simulink model "Controller_Exp"  (R2016a)
settings: Solver=ode4  StartTime=0.0  StopTime=Inf  FixedStep=Ts  RelTol=1e-3
undefined symbols (not defined in the file or in its folder): A_lpf_velocity, B1_lpf_velocity, B2_lpf_velocity, Calibration, commanded_u, GearOffsets, IMUTorsoOffsets, MedullaCommand, ResetDAQ, sample_time, TorsoCOMOffsets, Ts
libraries: xpcethercatlib x188, simulink x37, slrtlib x11, ControllerLibrary x2, dspswit3 x1
(part 4 of 4)

== system Controller_Exp/DAQ/DAQ_sub/Subsystem/EtherCATRobotMicrostrain/LegElmo_2R/Subsystem1/EnableControlWord ==
  Action Port : ActionPort  ActionType=case
  Constant : Constant  Value=15  OutDataTypeStr=uint16
  ControlWord : Outport
  wires:
  Constant/1 -> ControlWord/1

== system Controller_Exp/DAQ/DAQ_sub/Subsystem/EtherCATRobotMicrostrain/LegElmo_2R/Subsystem1/FaultReset ==
  Action Port : ActionPort  ActionType=case
  Constant : Constant  Value=128  OutDataTypeStr=uint16
  ControlWord : Outport
  wires:
  Constant/1 -> ControlWord/1

== system Controller_Exp/DAQ/DAQ_sub/Subsystem/EtherCATRobotMicrostrain/LegElmo_2R/Subsystem1/NothingControlWord ==
  Action Port : ActionPort  ActionType=default
  Constant : Constant  Value=0  OutDataTypeStr=uint16
  ControlWord : Outport
  wires:
  Constant/1 -> ControlWord/1

== system Controller_Exp/DAQ/DAQ_sub/Subsystem/EtherCATRobotMicrostrain/LegElmo_2R/Subsystem1/ShutdownControlWord ==
  Action Port : ActionPort  ActionType=case
  Constant : Constant  Value=6  OutDataTypeStr=uint16
  ControlWord : Outport
  wires:
  Constant/1 -> ControlWord/1

== matlab function Controller_Exp/DAQ/DAQ_sub/Subsystem/EstimateOrientation ==
  data: DeltaAngle input; Acceleration input; Status input; Sequence input; Reset input; Rk output; wk output; Rkm1 input; wkm1 input; Akm1 input; Ak output; Seqkm1 input; Seqk output; ValidStates output
function [Rk, wk, Ak, Seqk, ValidStates] = fcn(DeltaAngle,Acceleration,Status,Sequence,Reset,Rkm1,wkm1,Akm1,Seqkm1) %#codegen
    [Rk, wk, Ak, Seqk, ValidStates] = estimateOrientation(DeltaAngle,Acceleration,Rkm1,wkm1,Akm1,Status,Sequence,Seqkm1,Reset);
end

== matlab function Controller_Exp/DAQ/DAQ_sub/Subsystem/ComputeEulerAngles ==
  data: RkIn input; wk input; RCal input; Reset input; R0In input; ZYX output size=3; dZYX output size=3; Rk output; R0 output; YawRolloverIn input; YawRollover output
function [ZYX, dZYX, Rk, R0, YawRollover] = fcn(RkIn, wk, RCal, Reset, R0In, YawRolloverIn) %#codegen
    % Convert from IMU frame to robot frame and compute Euler angles. The
    % yaw angle is zeroed whenever (Reset) is true.
        
    if (Reset)
        % Compute the rotation matrix which zeroes the initial yaw
        qT0 = M_to_ZYX(RkIn*RCal);
        R0  = Rz(-qT0(1));
    else
        R0 = R0In;
    end
    
    % Transform from IMU to robot frame and zero initial yaw
    Rk = R0*RkIn*RCal;
    
    % Convert Rk to ZYX Euler angles
    ZYX = M_to_ZYX(Rk);
    
    % Unroll yaw
    YawRolloverCount = YawRolloverIn(1);
    PreviousYaw      = YawRolloverIn(2);
    CurrentYaw       = ZYX(1);
    YawRolloverCount = YawRolloverCount + getYawRollover(CurrentYaw, PreviousYaw);
    YawRollover      = [YawRolloverCount; CurrentYaw];
    ZYX(1)           = ZYX(1) + 2*pi*YawRolloverCount;
    
    % Compute Euler angle derivatives
    qzT = ZYX(1);
    qyT = ZYX(2);
    
    if cos(qyT)>1e-3
        dZYX = [0 -sin(qzT) cos(qzT)*cos(qyT); 0 cos(qzT) sin(qzT)*cos(qyT); 1 0 -sin(qyT)]\(R0*RkIn*wk);
    else
        dZYX = [0; 0; 0];
    end
end

function R = Rz(t)
    R = [cos(t) -sin(t) 0; sin(t) cos(t) 0; 0 0 1];
end

function Rollover = getYawRollover(CurrentYaw, PreviousYaw)
    % Determine if a rollover has occurred on yaw angle If a rollover is
    % detected, the output Rollover is either +1 or -1, depending on the
    % direction of the rollover.
  
    if (PreviousYaw>0 && CurrentYaw < (PreviousYaw-pi))
        Rollover = 1;
    elseif (PreviousYaw<0 && CurrentYaw > (PreviousYaw+pi))
        Rollover = -1;
    else
        Rollover = 0;
    end
end

== matlab function Controller_Exp/DAQ/DAQ_sub/Subsystem/EncoderFilters1/CheckAndFilterEncoder/Logic Filter ==
  data: q input; q_prev input; q_out output; q_good output; q_good_prev input
function [q_out,q_good] = fcn(q,q_prev,q_good_prev)
%#codegen

if abs(q - q_prev)*180/pi > 1
    q_out = max(min(q_good_prev,270/180*pi),90/180*pi);
    q_good = q_good_prev;
else
    q_out = q;
    q_good = q;
end

== matlab function Controller_Exp/DAQ/DAQ_sub/Subsystem/EncoderFilters1/CheckAndFilterEncoder/Velocity Filter/Logic Filter ==
  data: dq input; dq_prev input; dq_out output; dq_good output; dq_good_prev input
function [dq_out,dq_good] = fcn(dq,dq_prev,dq_good_prev)
%#codegen

if abs(dq - dq_prev)*180/pi > 20
    dq_out = max(min(dq_good_prev,200/180*pi),-200/180*pi);
    dq_good = dq_good_prev;
else
    dq_out = dq;
    dq_good = dq;
end

== matlab function Controller_Exp/DAQ/DAQ_sub/Subsystem/EncoderFilters/Filter/Median Filter ==
  data: q input; q_past input; q_out output
function q_out  = fcn(q,q_past)
%#codegen

q_all = [q,q_past];

if any(abs(diff(q_all))*180/pi > 1)
    q_out = median(q_all);
else
    q_out = q;
end

== matlab function Controller_Exp/DAQ/DAQ_sub/Subsystem/EncoderFilters/Filter/Velocity Filter/Median Filter ==
  data: dq input; dq_past input; dq_out output
function dq_out  = fcn(dq,dq_past)
%#codegen

dq_all = [dq,dq_past];

if any(abs(diff(dq_all))*180/pi > 20)
    dq_out = median(dq_all);
else
    dq_out = dq;
end

== matlab function Controller_Exp/DAQ/DAQ_sub/AdjustForCOMOffset ==
  data: q_in input; q output; TorsoCOMOffsets input
function q = fcn(q_in, TorsoCOMOffsets)
    %#codegen
    
    TorsoCOMRollOffset  = TorsoCOMOffsets(1)*pi/180;
    TorsoCOMPitchOffset = TorsoCOMOffsets(2)*pi/180;
    
    q = q_in;
    q(2)  = q(2)  + TorsoCOMRollOffset;
    q(10) = q(10) - TorsoCOMRollOffset;
    q(13) = q(13) + TorsoCOMRollOffset;
    
    q(3) = q(3) + TorsoCOMPitchOffset;
    q([4:9 11:12]) = q([4:9 11:12]) - TorsoCOMPitchOffset;
end

== matlab function Controller_Exp/DAQ/DAQ_sub/Subsystem/EtherCATRobotMicrostrain/ConvertAmpCurrent ==
  data: adc_value input; measuredCurrent output
function measuredCurrent = convert(adc_value)
    %#codegen

    measuredCurrent = (adc_value) * 60.0 / 8192;
end

== matlab function Controller_Exp/DAQ/DAQ_sub/Subsystem/EtherCATRobotMicrostrain/ConvertLogicVoltage ==
  data: adc_value input; logicVoltage output
function logicVoltage = convert(adc_value)
    %#codegen
    
    MEDULLA_ADC_MAX_VOLTS     = 2.70;
    MEDULLA_ADC_OFFSET_COUNTS = 172;
    
    logicVoltage = (adc_value - MEDULLA_ADC_OFFSET_COUNTS) * (MEDULLA_ADC_MAX_VOLTS/(4095.0))  * 6.0;
end

== matlab function Controller_Exp/DAQ/DAQ_sub/Subsystem/EtherCATRobotMicrostrain/ConvertMotorVoltage ==
  data: adc_value input; motorVoltage output
function motorVoltage = convert(adc_value)
    %#codegen
    
    MOTOR_VOLTAGE_C_OFFSET    = 1300.0;
    MOTOR_VOLTAGE_V_CAL       = 60.2;
    MOTOR_VOLTAGE_C_CAL       = 3600.0;
    
    motorVoltage = (adc_value - MOTOR_VOLTAGE_C_OFFSET)*MOTOR_VOLTAGE_V_CAL/(MOTOR_VOLTAGE_C_CAL-MOTOR_VOLTAGE_C_OFFSET);
end

== matlab function Controller_Exp/DAQ/DAQ_sub/Subsystem/EtherCATRobotMicrostrain/ConvertThermistors ==
  data: Temperatures output; adc_value input
function Temperatures  = convert(adc_value)
    %#codegen
    MEDULLA_ADC_MAX_VOLTS     = 2.70;
    MEDULLA_ADC_OFFSET_COUNTS = 172;
    
    processedADCValue = (adc_value - MEDULLA_ADC_OFFSET_COUNTS) * (MEDULLA_ADC_MAX_VOLTS/(4095.0));
    Temperatures = zeros(30,1); % 20141104
%     Temperatures = (1.0./( (1.0/298.15) + (1.0/3988.0)*log(4700.0./((3.26./processedADCValue) - 1.0)/10000))) - 273.15; %2015-12-17 DDA uncommend code
end

== matlab function Controller_Exp/DAQ/DAQ_sub/Subsystem/EtherCATRobotMicrostrain/EncodeSwitches ==
  data: Switches input; LimitSwitchesEncoded output
function LimitSwitchesEncoded = EncodeSwitches(Switches)
    LimitSwitchesVec     = uint32(Switches);
    LimitSwitchesEncoded = double(EncodeSwitches(LimitSwitchesVec));
end

== stateflow chart Controller_Exp/DAQ/DAQ_sub/Subsystem/EtherCATRobotMicrostrain/LegElmo_1L/Chart ==
  state Start1
    entry:
    ControlWordIndex = 0;
    EnableTargetTorque = 0;
    FaultDetected = 0;
  note: 2 = Medulla Run
  state Initialization
    state SwitchOnDisabled
      entry:
      ControlWordIndex = 1;
      Timeout = 0;
      EnableTargetTorque = 0;
      FaultDetected = 0;
      during:
      Timeout = Timeout + 1;
    state Fault
      entry:
      ControlWordIndex = 3;
      EnableTargetTorque = 0;
      Timeout = 0;
      FaultDetected = 0;
      during:
      Timeout = Timeout + 1;
      ControlWordIndex = 0;
    state ReadyToSwitchOn
      entry:
      ControlWordIndex = 2;
      Timeout = 0;
      EnableTargetTorque = 0;
      FaultDetected = 0;
      during:
      Timeout = Timeout + 1;
    (default) -> SwitchOnDisabled
    SwitchOnDisabled -> Fault [order 2] : [FaultMode == 1]
    Fault -> Fault [order 1] : [Timeout >=20]
    ReadyToSwitchOn -> SwitchOnDisabled [order 2] : [SwitchOnDisabledMode == 1]
    Fault -> SwitchOnDisabled [order 2] : [SwitchOnDisabledMode == 1]
    SwitchOnDisabled -> ReadyToSwitchOn [order 1] : [ReadyToSwitchOnMode == 1]
    ReadyToSwitchOn -> Fault [order 1] : [FaultMode == 1]
  state FaultRunning
    entry:
    ControlWordIndex = 1;
    EnableTargetTorque = 0;
    FaultDetected = 1;
  note: 5 = Error
  note: 4 = Halt
  state Running
    entry:
    FaultDetected = 0;
    ControlWordIndex = 2;
    EnableTargetTorque = 1;
  (default) -> Start1
  Start1 -> Initialization : [MedullaCommand == 2]
  FaultRunning -> Start1 : [MedullaCommand == 6]
  Initialization -> FaultRunning : [MedullaCommand == 4 || MedullaCommand == 5 ]
  Running -> FaultRunning [order 1] : [FaultMode == 1]
  Running -> FaultRunning [order 2] : [MedullaCommand == 4 || MedullaCommand == 5 ]
  ReadyToSwitchOn -> Running [order 3] : [EnabledMode == 1 && FaultMode == 0]
  data: SwitchOnDisabledMode input; EnabledMode input; ReadyToSwitchOnMode input; ControlWordIndex output; EnableTargetTorque output; Timeout local; FaultMode input; FaultDetected output; MedullaCommand input

== stateflow chart Controller_Exp/DAQ/DAQ_sub/Subsystem/EtherCATRobotMicrostrain/LegElmo_1R/Chart ==
  state Start1
    entry:
    ControlWordIndex = 0;
    EnableTargetTorque = 0;
    FaultDetected = 0;
  note: 2 = Medulla Run
  state Initialization
    state SwitchOnDisabled
      entry:
      ControlWordIndex = 1;
      Timeout = 0;
      EnableTargetTorque = 0;
      FaultDetected = 0;
      during:
      Timeout = Timeout + 1;
    state Fault
      entry:
      ControlWordIndex = 3;
      EnableTargetTorque = 0;
      Timeout = 0;
      FaultDetected = 0;
      during:
      Timeout = Timeout + 1;
      ControlWordIndex = 0;
    state ReadyToSwitchOn
      entry:
      ControlWordIndex = 2;
      Timeout = 0;
      EnableTargetTorque = 0;
      FaultDetected = 0;
      during:
      Timeout = Timeout + 1;
    (default) -> SwitchOnDisabled
    SwitchOnDisabled -> Fault [order 2] : [FaultMode == 1]
    Fault -> Fault [order 1] : [Timeout >=20]
    ReadyToSwitchOn -> SwitchOnDisabled [order 2] : [SwitchOnDisabledMode == 1]
    Fault -> SwitchOnDisabled [order 2] : [SwitchOnDisabledMode == 1]
    SwitchOnDisabled -> ReadyToSwitchOn [order 1] : [ReadyToSwitchOnMode == 1]
    ReadyToSwitchOn -> Fault [order 1] : [FaultMode == 1]
  state FaultRunning
    entry:
    ControlWordIndex = 1;
    EnableTargetTorque = 0;
    FaultDetected = 1;
  note: 5 = Error
  note: 4 = Halt
  state Running
    entry:
    FaultDetected = 0;
    ControlWordIndex = 2;
    EnableTargetTorque = 1;
  (default) -> Start1
  Start1 -> Initialization : [MedullaCommand == 2]
  FaultRunning -> Start1 : [MedullaCommand == 6]
  Initialization -> FaultRunning : [MedullaCommand == 4 || MedullaCommand == 5 ]
  Running -> FaultRunning [order 1] : [FaultMode == 1]
  Running -> FaultRunning [order 2] : [MedullaCommand == 4 || MedullaCommand == 5 ]
  ReadyToSwitchOn -> Running [order 3] : [EnabledMode == 1 && FaultMode == 0]
  data: SwitchOnDisabledMode input; EnabledMode input; ReadyToSwitchOnMode input; ControlWordIndex output; EnableTargetTorque output; Timeout local; FaultMode input; FaultDetected output; MedullaCommand input

== stateflow chart Controller_Exp/DAQ/DAQ_sub/Subsystem/EtherCATRobotMicrostrain/LegElmo_2L/Chart ==
  state Start1
    entry:
    ControlWordIndex = 0;
    EnableTargetTorque = 0;
    FaultDetected = 0;
  note: 2 = Medulla Run
  state Initialization
    state SwitchOnDisabled
      entry:
      ControlWordIndex = 1;
      Timeout = 0;
      EnableTargetTorque = 0;
      FaultDetected = 0;
      during:
      Timeout = Timeout + 1;
    state Fault
      entry:
      ControlWordIndex = 3;
      EnableTargetTorque = 0;
      Timeout = 0;
      FaultDetected = 0;
      during:
      Timeout = Timeout + 1;
      ControlWordIndex = 0;
    state ReadyToSwitchOn
      entry:
      ControlWordIndex = 2;
      Timeout = 0;
      EnableTargetTorque = 0;
      FaultDetected = 0;
      during:
      Timeout = Timeout + 1;
    (default) -> SwitchOnDisabled
    SwitchOnDisabled -> Fault [order 2] : [FaultMode == 1]
    Fault -> Fault [order 1] : [Timeout >=20]
    ReadyToSwitchOn -> SwitchOnDisabled [order 2] : [SwitchOnDisabledMode == 1]
    Fault -> SwitchOnDisabled [order 2] : [SwitchOnDisabledMode == 1]
    SwitchOnDisabled -> ReadyToSwitchOn [order 1] : [ReadyToSwitchOnMode == 1]
    ReadyToSwitchOn -> Fault [order 1] : [FaultMode == 1]
  state FaultRunning
    entry:
    ControlWordIndex = 1;
    EnableTargetTorque = 0;
    FaultDetected = 1;
  note: 5 = Error
  note: 4 = Halt
  state Running
    entry:
    FaultDetected = 0;
    ControlWordIndex = 2;
    EnableTargetTorque = 1;
  (default) -> Start1
  Start1 -> Initialization : [MedullaCommand == 2]
  FaultRunning -> Start1 : [MedullaCommand == 6]
  Initialization -> FaultRunning : [MedullaCommand == 4 || MedullaCommand == 5 ]
  Running -> FaultRunning [order 1] : [FaultMode == 1]
  Running -> FaultRunning [order 2] : [MedullaCommand == 4 || MedullaCommand == 5 ]
  ReadyToSwitchOn -> Running [order 3] : [EnabledMode == 1 && FaultMode == 0]
  data: SwitchOnDisabledMode input; EnabledMode input; ReadyToSwitchOnMode input; ControlWordIndex output; EnableTargetTorque output; Timeout local; FaultMode input; FaultDetected output; MedullaCommand input

== stateflow chart Controller_Exp/DAQ/DAQ_sub/Subsystem/EtherCATRobotMicrostrain/LegElmo_2R/Chart ==
  state Start1
    entry:
    ControlWordIndex = 0;
    EnableTargetTorque = 0;
    FaultDetected = 0;
  note: 2 = Medulla Run
  state Initialization
    state SwitchOnDisabled
      entry:
      ControlWordIndex = 1;
      Timeout = 0;
      EnableTargetTorque = 0;
      FaultDetected = 0;
      during:
      Timeout = Timeout + 1;
    state Fault
      entry:
      ControlWordIndex = 3;
      EnableTargetTorque = 0;
      Timeout = 0;
      FaultDetected = 0;
      during:
      Timeout = Timeout + 1;
      ControlWordIndex = 0;
    state ReadyToSwitchOn
      entry:
      ControlWordIndex = 2;
      Timeout = 0;
      EnableTargetTorque = 0;
      FaultDetected = 0;
      during:
      Timeout = Timeout + 1;
    (default) -> SwitchOnDisabled
    SwitchOnDisabled -> Fault [order 2] : [FaultMode == 1]
    Fault -> Fault [order 1] : [Timeout >=20]
    ReadyToSwitchOn -> SwitchOnDisabled [order 2] : [SwitchOnDisabledMode == 1]
    Fault -> SwitchOnDisabled [order 2] : [SwitchOnDisabledMode == 1]
    SwitchOnDisabled -> ReadyToSwitchOn [order 1] : [ReadyToSwitchOnMode == 1]
    ReadyToSwitchOn -> Fault [order 1] : [FaultMode == 1]
  state FaultRunning
    entry:
    ControlWordIndex = 1;
    EnableTargetTorque = 0;
    FaultDetected = 1;
  note: 5 = Error
  note: 4 = Halt
  state Running
    entry:
    FaultDetected = 0;
    ControlWordIndex = 2;
    EnableTargetTorque = 1;
  (default) -> Start1
  Start1 -> Initialization : [MedullaCommand == 2]
  FaultRunning -> Start1 : [MedullaCommand == 6]
  Initialization -> FaultRunning : [MedullaCommand == 4 || MedullaCommand == 5 ]
  Running -> FaultRunning [order 1] : [FaultMode == 1]
  Running -> FaultRunning [order 2] : [MedullaCommand == 4 || MedullaCommand == 5 ]
  ReadyToSwitchOn -> Running [order 3] : [EnabledMode == 1 && FaultMode == 0]
  data: SwitchOnDisabledMode input; EnabledMode input; ReadyToSwitchOnMode input; ControlWordIndex output; EnableTargetTorque output; Timeout local; FaultMode input; FaultDetected output; MedullaCommand input

== matlab function Controller_Exp/DAQ/DAQ_sub/Subsystem/ZeroingLegs ==
  data: u input; u_zeroed output
function u_zeroed = ZeroingLegs(u)

% leg_motor_1R_torque_cmd = u(1);
% leg_motor_2R_torque_cmd = u(2);
% hip_motor_3R_torque_cmd = u(3);
% leg_motor_1L_torque_cmd = u(4);
% leg_motor_2L_torque_cmd = u(5);
% hip_motor_3L_torque_cmd = u(6);

u_zeroed = [0;
            0;
            u(3);
            0;
            0;
            u(6)];

end

== matlab function Controller_Exp/DAQ/DAQ_sub/Subsystem/calibrate ==
  data: Calibration input; AbsEncoders input; IncEncoders input; IncEncodersPrev input; AbsAngle output; Reset input; IncAngle output; RolloverIn input; Rollover output; IncCalTickIn input; IncCalTick output
function [AbsAngle, IncAngle, Rollover, IncCalTick] = calibrate(Calibration,AbsEncoders,IncEncoders,IncEncodersPrev,Reset,RolloverIn,IncCalTickIn)
    %#codegen
    [AbsAngle, IncAngle, Rollover, IncCalTick] = calibrateEncoders_ATRIAS(Calibration,AbsEncoders,IncEncoders,IncEncodersPrev,Reset,RolloverIn,IncCalTickIn);
end

== matlab function Controller_Exp/DAQ/DAQ_sub/Subsystem/convert_mtr_current_to_pwm ==
  data: params input; u input; y output; Reset input
function y = convert_to_pwm(params,u,Reset)
%#codegen
%This function takes motor torque command inputs and outputs
%pwm commands (for the Medulla) in UMich convention

y = zeros(6,1);

if (Reset)
    return
end

%The inputs, which are commanded motor torques 
leg_motor_1R_torque_cmd = u(1);
leg_motor_2R_torque_cmd = u(2);
hip_motor_3R_torque_cmd = u(3);
leg_motor_1L_torque_cmd = u(4);
leg_motor_2L_torque_cmd = u(5);
hip_motor_3L_torque_cmd = u(6);

%Parameters determined experimentally at U Mich
UMich_LEFT_MOTOR_HIP_DIRECTION = params(1); %The direction for the left hip motor. (UMich convention)
UMich_RIGHT_MOTOR_HIP_DIRECTION = params(2); %The direction for the right hip motor. (UMich convention)

% The parameters, from http://code.google.com/p/atrias/source/browse/robot_definitions/
%From robot_invariant_defs.h
MTR_MAX_COUNT = params(3); %The maximum commanded amplifier value. This is the maximum value sent to the Medullas for the amplifier command.
%From biped2_variant_defs.h
MTR_MAX_TORQUE = params(4); %Maximum motor torque for scaling
MTR_HIP_MAX_TORQUE = params(5); %Maximum hip motor torque for scaling
%From leg3_definitions.h (corresponds to our left leg)
%(Note that A=shin and B=thigh for OSU convention)
LEG3_MOTOR_A_DIRECTION = params(6);
LEG3_MOTOR_B_DIRECTION = params(7);
%From leg4_definitions.h (corresponds to our right leg)
%(Note that A=shin and B=thigh for OSU convention)
LEG4_MOTOR_A_DIRECTION = params(8);
LEG4_MOTOR_B_DIRECTION = params(9);

leg_torque_to_pwm = MTR_MAX_COUNT/MTR_MAX_TORQUE;
hip_torque_to_pwm = MTR_MAX_COUNT/MTR_HIP_MAX_TORQUE;

%Convert leg_motor_1L_torque_cmd
leg_motor_1L_direction = LEG3_MOTOR_A_DIRECTION;
y(1) = motor_torque_to_pwm(leg_motor_1L_direction,leg_torque_to_pwm,leg_motor_1L_torque_cmd);

%Convert leg_motor_2L_torque_cmd
leg_motor_2L_direction = LEG3_MOTOR_B_DIRECTION;
y(2) = motor_torque_to_pwm(leg_motor_2L_direction,leg_torque_to_pwm,leg_motor_2L_torque_cmd);

%Convert leg_motor_1R_torque_cmd
leg_motor_1R_direction = LEG4_MOTOR_A_DIRECTION;
y(3) = motor_torque_to_pwm(leg_motor_1R_direction,leg_torque_to_pwm,leg_motor_1R_torque_cmd);

%Convert leg_motor_2R_torque_cmd
leg_motor_2R_direction = LEG4_MOTOR_B_DIRECTION;
y(4) = motor_torque_to_pwm(leg_motor_2R_direction,leg_torque_to_pwm,leg_motor_2R_torque_cmd);

%Convert hip_motor_3R_torque_cmd
hip_motor_3R_direction = UMich_RIGHT_MOTOR_HIP_DIRECTION; %Verified experimentally
y(5) = motor_torque_to_pwm(hip_motor_3R_direction,hip_torque_to_pwm,hip_motor_3R_torque_cmd);

%Convert hip_motor_3L_torque_cmd
hip_motor_3L_direction = UMich_LEFT_MOTOR_HIP_DIRECTION; %Verified experimentally
y(6) = motor_torque_to_pwm(hip_motor_3L_direction,hip_torque_to_pwm,hip_motor_3L_torque_cmd);

end

function motor_pwm = motor_torque_to_pwm(motor_direction,torque_to_pwm_const,motor_torque_cmd)
   motor_pwm = motor_direction*torque_to_pwm_const*motor_torque_cmd;
end

== matlab function Controller_Exp/DAQ/DAQ_sub/StateEstimator/GeneralizedCoordinates ==
  data: EncoderAngles input; EncoderVelocities input; q_clean output; IMUAngles input; IMUVelocities input; UseMotorIncEncoders input; UseIMU input; dq_clean output; IMUTorsoOffset input; GearOffset input; Reset input
function [q_clean, dq_clean] = coords(EncoderAngles, EncoderVelocities, IMUAngles, IMUVelocities, UseMotorIncEncoders, UseIMU, IMUTorsoOffset, GearOffset, Reset)
    %#codegen
    
    % q_clean =
    %  [qzT; qyT; qxT; q1R; q2R; q1L; q2L; qgr1R; qgr2R; q3R; qgr1L; qgr2L; q3L];
    %
    % EncoderAngles = 
    %  [Leg1R; Leg2R; Leg1L; Leg2L; Motor1R; Motor2R; Motor1L; Motor2L; Hip3R; Hip3L; ...   % ABSOLUTE ENCODERS
    %   Inc1R; Inc2R; Inc1L; Inc2L; Inc3R; Inc3L; Boom; Boom; Boom]                         % INCREMENTAL ENCODERS
    
    if (Reset)
        q_clean  = zeros(13,1);
        dq_clean = zeros(13,1);
    else 
        q_clean  = EncoderAngles([17:19 1:6 15 7:8 16]);
        dq_clean = EncoderVelocities([17:19 1:6 15 7:8 16]);
        
        % DDA 2015-10-13
        % Use hip abs encoder. The left inc encoder drift. Still use inc
        % for velocity because the abs velocity is too noisy. Otherwise,
        % add a more restrict filter for that.
        q_clean([10 13]) = EncoderAngles([9 10]);
%         dq_clean([10 13]) = EncoderVelocities([9 10]);
        
        if (UseMotorIncEncoders)
            if 0
                q_clean([8:9 11:12])  = EncoderAngles(11:14)/50;
                dq_clean([8:9 11:12]) = EncoderVelocities(11:14)/50;
                
            elseif 0
                % BGB 2014-08-29
                % The incremental encoder on q1L was destroyed in the 60V
                % power fault event, so it cannot be used until it is
                % replaced.
                q_clean([8:9 12])  = EncoderAngles([11:12 14])/50;
                dq_clean([8:9 12]) = EncoderVelocities([11:12 14])/50;

            elseif 0
                % BGB 2015-02-05
                % Perhaps the harmonic drive is bad? We are seeing drift in
                % the 2L incremental motor encoder.
                q_clean(8:9)  = EncoderAngles(11:12)/50;
                dq_clean(8:9) = EncoderVelocities(11:12)/50;
                
            else
                % DDA 2015-12-17
                % Use non incremental encoder, they will be read from Elmo
                % in near future
            end
        end
        
        % Add offset to gear angles to allow zeroing of spring deflections.
        q_clean([8:9 11:12]) = q_clean([8:9 11:12]) + GearOffset*pi/180;
        
        if (UseIMU)
            q_clean(1:3)  = IMUAngles + [0; IMUTorsoOffset]*pi/180;
            dq_clean(1:3) = IMUVelocities;
        end
    end
end

== matlab function Controller_Exp/DAQ/DAQ_sub/SAFETY ==
  data: MotorCurrentCommand input; MotorCurrentCommandSafe output; MedullaCommand input; RequestSoftStop input; q input; dq input; SafetyCountIn input; MedullaCommandSafe output; SafetyState output; SafetyCountOut output
function [MotorCurrentCommandSafe, MedullaCommandSafe, SafetyState, SafetyCountOut] = SafetyCheck(MotorCurrentCommand, MedullaCommand, RequestSoftStop, q, dq, SafetyCountIn)
    SelectBasicLimits = 5;
    [MotorCurrentCommandSafe, MedullaCommandSafe, SafetyState, SafetyCountOut] = MARLOSafety_ATRIAS(MotorCurrentCommand, MedullaCommand, RequestSoftStop, q, dq, SafetyCountIn, SelectBasicLimits);
	
end
